simulink model "test"  (R2017a)
settings: Solver=VariableStepAuto  StartTime=0.0  StopTime=10.0  RelTol=1e-3
settings Model: Creator=zdw7287  LastModifiedBy=zdw7287

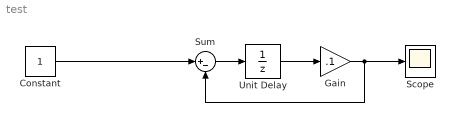
== system test ==
  Constant : Constant
  Gain : Gain  Gain=.1
  Scope : Scope
  Sum : Sum  Inputs=|+-
  Unit Delay : UnitDelay  SampleTime=-1
  wires:
  Constant/1 -> Sum/1
  Sum/1 -> Unit Delay/1
  Gain/1 -> Scope/1, Sum/2
  Unit Delay/1 -> Gain/1
